simulink model "system_control"  (R2021a)
settings: Solver=FixedStepAuto  StartTime=0.0  StopTime=60  FixedStep=0.02  RelTol=1e-3
undefined symbols (not defined in the file): alpha, tau_d, v, yaw
libraries: simulink x2
(part 1 of 2)
settings Model: Creator=frede  LastModifiedBy=frede
settings DataIOCC: ReturnWorkspaceOutputs=off

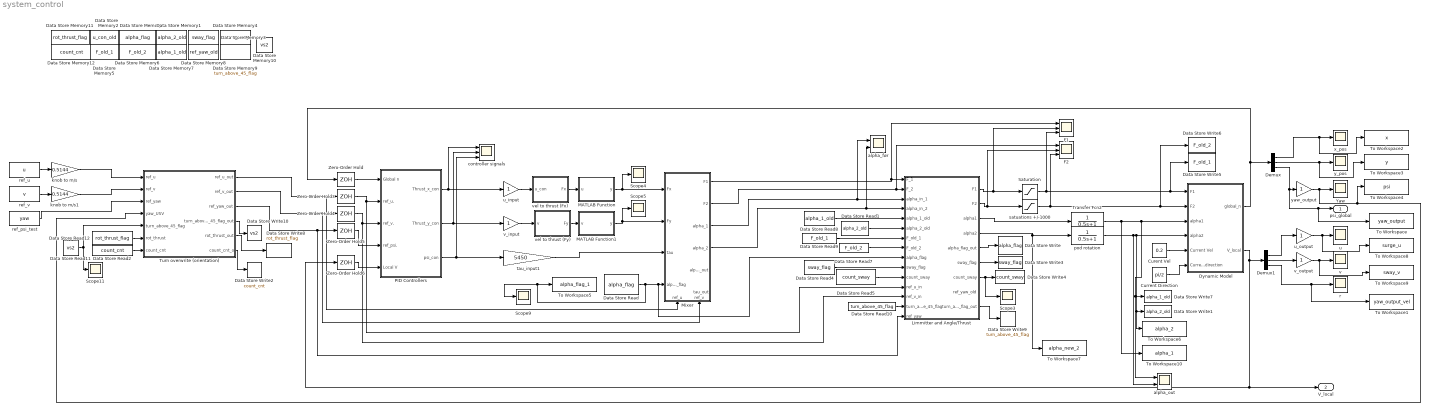
== system system_control ==
  Curent Vel : Constant  Value=0.2
  Current Direction : Constant  Value=pi/2
  Data Store Memory : DataStoreMemory  DataStoreName=alpha_flag  ReadBeforeWriteMsg=warning  WriteAfterWriteMsg=warning  WriteAfterReadMsg=warning  ShowAdditionalParam=off
  Data Store Memory1 : DataStoreMemory  DataStoreName=alpha_2_old  ReadBeforeWriteMsg=warning  WriteAfterWriteMsg=warning  WriteAfterReadMsg=warning  ShowAdditionalParam=off
  Data Store Memory10 : DataStoreMemory  DataStoreName=vs2  ReadBeforeWriteMsg=warning  WriteAfterWriteMsg=warning  WriteAfterReadMsg=warning  ShowAdditionalParam=off
  Data Store Memory11 : DataStoreMemory  DataStoreName=rot_thrust_flag  ReadBeforeWriteMsg=warning  WriteAfterWriteMsg=warning  WriteAfterReadMsg=warning  ShowAdditionalParam=off
  Data Store Memory12 : DataStoreMemory  DataStoreName=count_cnt  ReadBeforeWriteMsg=warning  WriteAfterWriteMsg=warning  WriteAfterReadMsg=warning  ShowAdditionalParam=off
  Data Store Memory2 : DataStoreMemory  DataStoreName=u_con_old  ReadBeforeWriteMsg=warning  WriteAfterWriteMsg=warning  WriteAfterReadMsg=warning  ShowAdditionalParam=off
  Data Store Memory3 : DataStoreMemory  DataStoreName=sway_flag  ReadBeforeWriteMsg=warning  WriteAfterWriteMsg=warning  WriteAfterReadMsg=warning  ShowAdditionalParam=off
  Data Store Memory4 : DataStoreMemory  DataStoreName=count_sway  ReadBeforeWriteMsg=warning  WriteAfterWriteMsg=warning  WriteAfterReadMsg=warning  ShowAdditionalParam=off
  Data Store Memory5 : DataStoreMemory  DataStoreName=F_old_1  ReadBeforeWriteMsg=warning  WriteAfterWriteMsg=warning  WriteAfterReadMsg=warning  ShowAdditionalParam=off
  Data Store Memory6 : DataStoreMemory  DataStoreName=F_old_2  ReadBeforeWriteMsg=warning  WriteAfterWriteMsg=warning  WriteAfterReadMsg=warning  ShowAdditionalParam=off
  Data Store Memory7 : DataStoreMemory  DataStoreName=alpha_1_old  ReadBeforeWriteMsg=warning  WriteAfterWriteMsg=warning  WriteAfterReadMsg=warning  ShowAdditionalParam=off
  Data Store Memory8 : DataStoreMemory  DataStoreName=ref_yaw_old  ReadBeforeWriteMsg=warning  WriteAfterWriteMsg=warning  WriteAfterReadMsg=warning  ShowAdditionalParam=off
  Data Store Memory9 : DataStoreMemory  DataStoreName=turn_above_45_flag  ReadBeforeWriteMsg=warning  WriteAfterWriteMsg=warning  WriteAfterReadMsg=warning  ShowAdditionalParam=off
  Data Store Read : DataStoreRead  DataStoreName=alpha_flag  IndexOptions=Index vector (dialog)  Indices=1  OutputSizes=1
  Data Store Read1 : DataStoreRead  DataStoreName=alpha_2_old  IndexOptions=Index vector (dialog)  Indices=1  OutputSizes=1
  Data Store Read10 : DataStoreRead  DataStoreName=turn_above_45_flag  IndexOptions=Index vector (dialog)  Indices=1  OutputSizes=1
  Data Store Read11 : DataStoreRead  DataStoreName=vs2  IndexOptions=Index vector (dialog)  Indices=1  OutputSizes=1
  Data Store Read12 : DataStoreRead  DataStoreName=rot_thrust_flag  IndexOptions=Index vector (dialog)  Indices=1  OutputSizes=1
  Data Store Read2 : DataStoreRead  DataStoreName=count_cnt  IndexOptions=Index vector (dialog)  Indices=1  OutputSizes=1
  Data Store Read4 : DataStoreRead  DataStoreName=sway_flag  IndexOptions=Index vector (dialog)  Indices=1  OutputSizes=1
  Data Store Read5 : DataStoreRead  DataStoreName=count_sway  IndexOptions=Index vector (dialog)  Indices=1  OutputSizes=1
  Data Store Read7 : DataStoreRead  DataStoreName=F_old_2  IndexOptions=Index vector (dialog)  Indices=1  OutputSizes=1
  Data Store Read8 : DataStoreRead  DataStoreName=alpha_1_old  IndexOptions=Index vector (dialog)  Indices=1  OutputSizes=1
  Data Store Read9 : DataStoreRead  DataStoreName=F_old_1  IndexOptions=Index vector (dialog)  Indices=1  OutputSizes=1
  Data Store Write : DataStoreWrite  DataStoreName=alpha_flag  IndexOptions=Index vector (dialog)  Indices=1  OutputSizes=1
  Data Store Write1 : DataStoreWrite  DataStoreName=alpha_2_old  IndexOptions=Index vector (dialog)  Indices=1  OutputSizes=1
  Data Store Write10 : DataStoreWrite  DataStoreName=vs2  IndexOptions=Index vector (dialog)  Indices=1  OutputSizes=1
  Data Store Write2 : DataStoreWrite  DataStoreName=count_cnt  IndexOptions=Index vector (dialog)  Indices=1  OutputSizes=1
  Data Store Write3 : DataStoreWrite  DataStoreName=sway_flag  IndexOptions=Index vector (dialog)  Indices=1  OutputSizes=1
  Data Store Write4 : DataStoreWrite  DataStoreName=count_sway  IndexOptions=Index vector (dialog)  Indices=1  OutputSizes=1
  Data Store Write5 : DataStoreWrite  DataStoreName=F_old_1  IndexOptions=Index vector (dialog)  Indices=1  OutputSizes=1
  Data Store Write6 : DataStoreWrite  DataStoreName=F_old_2  IndexOptions=Index vector (dialog)  Indices=1  OutputSizes=1
  Data Store Write7 : DataStoreWrite  DataStoreName=alpha_1_old  IndexOptions=Index vector (dialog)  Indices=1  OutputSizes=1
  Data Store Write8 : DataStoreWrite  DataStoreName=rot_thrust_flag  IndexOptions=Index vector (dialog)  Indices=1  OutputSizes=1
  Data Store Write9 : DataStoreWrite  DataStoreName=turn_above_45_flag  IndexOptions=Index vector (dialog)  Indices=1  OutputSizes=1
  Demux : Demux  Outputs=3
  Demux1 : Demux  Outputs=3
  Dynamic Model : Subsystem
  F1 : Scope  NumInputPorts=3
  F2 : Scope  NumInputPorts=3
  "Limmitter and Angle/Thrust " : MATLAB Function  TreatAsAtomicUnit=on
  MATLAB Function : MATLAB Function  TreatAsAtomicUnit=on
  MATLAB Function1 : MATLAB Function  TreatAsAtomicUnit=on
  Mixer : Subsystem
      settings: PortSchema="{\"entries\":[{\"content\":{\"sides\":[{\"content\":{\"connectorIds\":[\"In1\",\"In2\",\"In3\",\"In4\"]},\"type\":\"ConnectorPlacement.EquallySpacedRectSide\",\"uuid\":\"7188d02b-cfcc-47db-af94-18894173419c\"},{\"content\":{\"connectorIds\":[\"Out1\",\"Out2\",\"Out3\",\"Out4\",\"Out5\",\"Out6\"],\"side\":\"RIGHT\"},\"type\":\"ConnectorPlacement.EquallySpacedRectSide\",\"uuid\":\"02945fdb-bbe4-4a20-85bf-b896b72802e6\"},{\"content\":{\"connectorIds\":[],\"side\":\"TOP\"},\"type\":\"ConnectorPlacement.EquallySpacedRectSide\",\"uuid\":\"f10c450a-087c-46ba-bf6c-a28873fc7004\"},{\"content\":{\"connectorIds\":[\"In5\",\"In6\"],\"side\":\"BOTTOM\"},\"type\":\"ConnectorPlacement.EquallySpacedRectSide\",\"uuid\":\"e6b9d579-da5b-4e58-b3fd-82de45e53b4e\"}]},\"type\":\"ConnectorPlacement.EquallySpacedConnector\",\"uuid\":\"11fe65e6-3ea5-4662-a95f-67184bab7731\"}],\"packageUris\":[\"http://schema.mathworks.com/mf0/Connector/R2020b\"],\"version\":\"1.0\"}"
  PID Controllers : Subsystem
  Saturation : Saturate  UpperLimit=1000  LowerLimit=-1000
  Scope{3..5,9,11} (5 alike) : Scope
  To Workspace : ToWorkspace  VariableName=yaw_output  SaveFormat=Timeseries  SampleTime=-1
  To Workspace1 : ToWorkspace  VariableName=yaw_output_vel  SaveFormat=Timeseries  SampleTime=-1
  To Workspace10 : ToWorkspace  VariableName=alpha_1  SaveFormat=Timeseries  SampleTime=-1
  To Workspace2 : ToWorkspace  VariableName=x  SaveFormat=Timeseries  SampleTime=-1
  To Workspace3 : ToWorkspace  VariableName=y  SaveFormat=Timeseries  SampleTime=-1
  To Workspace4 : ToWorkspace  VariableName=psi  SaveFormat=Timeseries  SampleTime=-1
  To Workspace5 : ToWorkspace  VariableName=alpha_flag_1  SaveFormat=Timeseries  SampleTime=-1
  To Workspace6 : ToWorkspace  VariableName=alpha_2  SaveFormat=Timeseries  SampleTime=-1
  To Workspace7 : ToWorkspace  VariableName=alpha_new_2  SaveFormat=Timeseries  SampleTime=-1
  To Workspace8 : ToWorkspace  VariableName=surge_u  SaveFormat=Timeseries  SampleTime=-1
  To Workspace9 : ToWorkspace  VariableName=sway_v  SaveFormat=Timeseries  SampleTime=-1
  Transfer Fcn2 : TransferFcn  Denominator=[0.5 1]
  Turn overwrite (orientation) : MATLAB Function  TreatAsAtomicUnit=on
  Yaw : Scope
  Zero-Order Hold{,3..6} (5 alike) : ZeroOrderHold  SampleTime=1/10
  alpha_før : Scope  NumInputPorts=2
  alpha_out : Scope  NumInputPorts=2
  controller signals : Scope  NumInputPorts=3
  knob to m/s : Gain  Gain=0.5144
  knob to m/s1 : Gain  Gain=0.5144
  pod rotation : TransferFcn  Denominator=[0.5 1]
  r : Scope
  ref_psi_test : Constant  Value=yaw
  ref_u : Constant  Value=u
  ref_v : Constant  Value=v
  "satuations +/-1000 " : Saturate  UpperLimit=1000  LowerLimit=-1000
  tau_input1 : Gain  Gain=5450
  u : Scope
  u_input : Gain
  u_output : Gain
  v : Scope
  v_input : Gain
  v_output : Gain
  vel to thrust (Fx) : MATLAB Function  TreatAsAtomicUnit=on
  vel to thrust (Fy) : MATLAB Function  TreatAsAtomicUnit=on
  x_pos : Scope
  y_pos : Scope
  yaw_output : Gain
  psi_global : Outport
  V_local : Outport  Port=2
  wires:
  vel to thrust (Fx)/1(Fx) -> MATLAB Function/1(u)
  Demux1/3 -> r/1, To Workspace1/1
  "Limmitter and Angle/Thrust "/2(F2) -> "satuations +/-1000 "/1, F2/2
  Mixer/1(F1) -> F1/1, "Limmitter and Angle/Thrust "/1(F_1)
  v_input/1 -> vel to thrust (Fy)/1(v)
  Mixer/4(alpha_2) -> alpha_før/2, "Limmitter and Angle/Thrust "/4(alpha_in_2)
  Demux1/2 -> v_output/1
  Mixer/2(F2) -> F2/1, "Limmitter and Angle/Thrust "/2(F_2)
  "Limmitter and Angle/Thrust "/3(alpha1) -> Transfer Fcn2/1
  u_input/1 -> vel to thrust (Fx)/1(u_con)
  MATLAB Function1/1(y) -> Scope5/1, Mixer/2(Fy)
  Mixer/3(alpha_1) -> alpha_før/1, "Limmitter and Angle/Thrust "/3(alpha_in_1)
  "Limmitter and Angle/Thrust "/1(F1) -> F1/2, Saturation/1
  Demux/2 -> To Workspace3/1, y_pos/1
  "satuations +/-1000 "/1 -> Data Store Write6/1, Dynamic Model/2(F2), F2/3
  Demux1/1 -> u_output/1
  Transfer Fcn2/1 -> To Workspace10/1, Data Store Write7/1, alpha_out/1, Dynamic Model/3(alpha1)
  Dynamic Model/1(global_n) -> Zero-Order Hold/1, Demux/1
  "Limmitter and Angle/Thrust "/4(alpha2) -> To Workspace7/1, pod rotation/1
  Demux/1 -> To Workspace2/1, x_pos/1
  v_output/1 -> To Workspace9/1, v/1
  Saturation/1 -> Data Store Write5/1, Dynamic Model/1(F1), F1/3
  ref_v/1 -> knob to m/s1/1
  Demux/3 -> yaw_output/1, To Workspace/1, psi_global/1
  MATLAB Function/1(y) -> Mixer/1(Fx), Scope4/1
  yaw_output/1 -> Yaw/1, Turn overwrite (orientation)/4(yaw_USV), To Workspace4/1
  vel to thrust (Fy)/1(Fy) -> MATLAB Function1/1(v)
  Turn overwrite (orientation)/3(ref_yaw_out) -> "Limmitter and Angle/Thrust "/15(ref_yaw), Zero-Order Hold5/1
  Curent Vel/1 -> Dynamic Model/5(Current Vel)
  Current Direction/1 -> Dynamic Model/6(Current direction)
  ref_u/1 -> knob to m/s/1
  Turn overwrite (orientation)/2(ref_v_out) -> Zero-Order Hold4/1, Mixer/6(ref_v)
  "Limmitter and Angle/Thrust "/5(alpha_flag_out) -> Data Store Write/1
  Data Store Read1/1 -> "Limmitter and Angle/Thrust "/6(alpha_2_old)
  Data Store Read/1 -> Scope9/1, To Workspace5/1, "Limmitter and Angle/Thrust "/9(alpha_flag), Mixer/4(alpha_flag)
  Zero-Order Hold/1 -> PID Controllers/1(Global n)
  Turn overwrite (orientation)/1(ref_u_out) -> Zero-Order Hold3/1, Mixer/5(ref_u)
  Dynamic Model/2(V_local) -> V_local/1, Zero-Order Hold6/1, Demux1/1
  Zero-Order Hold3/1 -> "Limmitter and Angle/Thrust "/12(ref_u_in), PID Controllers/2(ref_u.)
  Zero-Order Hold4/1 -> "Limmitter and Angle/Thrust "/13(ref_v_in), PID Controllers/3(ref_v.)
  Zero-Order Hold5/1 -> PID Controllers/4(ref_psi.)
  Zero-Order Hold6/1 -> PID Controllers/5(Local V)
  "Limmitter and Angle/Thrust "/6(sway_flag) -> Data Store Write3/1
  Data Store Read5/1 -> "Limmitter and Angle/Thrust "/11("count_sway ")
  tau_input1/1 -> Mixer/3(tau)
  Data Store Read8/1 -> "Limmitter and Angle/Thrust "/5(alpha_1_old)
  Data Store Read7/1 -> "Limmitter and Angle/Thrust "/8(F_old_2)
  Data Store Read9/1 -> "Limmitter and Angle/Thrust "/7(F_old_1)
  Data Store Read4/1 -> "Limmitter and Angle/Thrust "/10("sway_flag ")
  "Limmitter and Angle/Thrust "/7(count_sway) -> Scope3/1, Data Store Write4/1
  Data Store Read10/1 -> "Limmitter and Angle/Thrust "/14(turn_above_45_flag)
  "Limmitter and Angle/Thrust "/9(turn_above_45_flag_out) -> Data Store Write9/1
  Turn overwrite (orientation)/4(turn_above_45_flag_out) -> Data Store Write10/1
  Data Store Read11/1 -> Turn overwrite (orientation)/5(turn_above_45_flag), Scope11/1
  PID Controllers/2(Thrust_y_con) -> v_input/1, controller signals/2
  PID Controllers/1(Thrust_x_con) -> u_input/1, controller signals/1
  PID Controllers/3(psi_con) -> tau_input1/1, controller signals/3
  Data Store Read12/1 -> Turn overwrite (orientation)/6(rot_thrust)
  Turn overwrite (orientation)/5(rot_thrust_out) -> Data Store Write8/1
  knob to m/s/1 -> Turn overwrite (orientation)/1(ref_u)
  knob to m/s1/1 -> Turn overwrite (orientation)/2(ref_v)
  ref_psi_test/1 -> Turn overwrite (orientation)/3(ref_yaw)
  pod rotation/1 -> Dynamic Model/4(alpha2), To Workspace6/1, Data Store Write1/1, alpha_out/2
  Turn overwrite (orientation)/6(count_cnt_o) -> Data Store Write2/1
  Data Store Read2/1 -> Turn overwrite (orientation)/7(count_cnt)
  u_output/1 -> To Workspace8/1, u/1

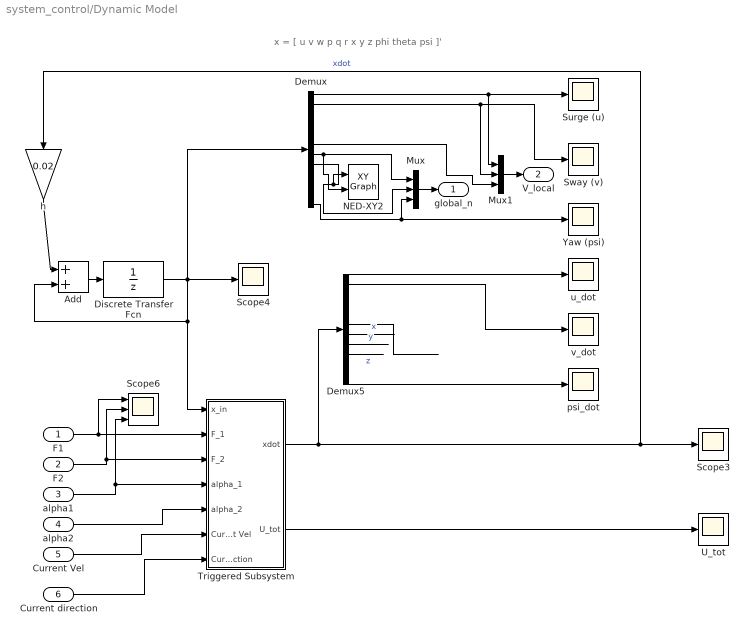
== system system_control/Dynamic Model ==
  note: x = [ u v w p q r x y z phi theta psi ]'
  F1 : Inport
  F2 : Inport  Port=2
  alpha1 : Inport  Port=3
  alpha2 : Inport  Port=4
  Current Vel : Inport  Port=5
  Current direction : Inport  Port=6
  Add : Sum
  Demux : Demux  Outputs=12
  Demux5 : Demux  Outputs=12
  Discrete Transfer Fcn : DiscreteTransferFcn  Denominator=[ 1 0]  SampleTime=0.02
  Mux : Mux  Inputs=3
  Mux1 : Mux  Inputs=3
  NED-XY2 : simulink/Sinks/XY Graph  xmin=-10  xmax=100  ymin=-10  ymax=100  st=-1
  Scope3 : Scope
  Scope4 : Scope
  Scope6 : Scope  NumInputPorts=3
  Surge (u) : Scope
  Sway (v) : Scope
  Triggered Subsystem : Subsystem  TreatAsAtomicUnit=on
  U_tot : Scope
  Yaw (psi) : Scope
  h : Gain  Gain=0.02
  psi_dot : Scope
  u_dot : Scope
  v_dot : Scope
  global_n : Outport
  V_local : Outport  Port=2
  wires:
  F1/1 -> Scope6/1, Triggered Subsystem/2(F_1)
  F2/1 -> Scope6/2, Triggered Subsystem/3(F_2)
  alpha1/1 -> Scope6/3, Triggered Subsystem/4(alpha_1)
  alpha2/1 -> Triggered Subsystem/5(alpha_2)
  h/1 -> Add/1
  Add/1 -> Discrete Transfer Fcn/1
  Triggered Subsystem/1(xdot) -> Demux5/1, Scope3/1, h/1  "xdot"
  Triggered Subsystem/2(U_tot) -> U_tot/1
  Demux/8 -> Mux/2, NED-XY2/1
  Demux/7 -> NED-XY2/2, Mux/1
  Discrete Transfer Fcn/1 -> Scope4/1, Demux/1, Add/2, Triggered Subsystem/1(x_in)
  Demux/1 -> Surge (u)/1, Mux1/1
  Demux/12 -> Mux/3, Yaw (psi)/1
  Demux/2 -> Mux1/2, Sway (v)/1
  Mux/1 -> global_n/1
  Demux5/12 -> psi_dot/1
  Demux5/2 -> v_dot/1
  Demux5/1 -> u_dot/1
  Demux5/9 -> ?  "z"
  Demux5/7 -> ?  "x"
  Demux5/8 -> ?  "y"
  Mux1/1 -> V_local/1
  Demux5/6 -> ?
  Demux/6 -> Mux1/3
  Current Vel/1 -> Triggered Subsystem/6(Current Vel)
  Current direction/1 -> Triggered Subsystem/7(Current Direction)

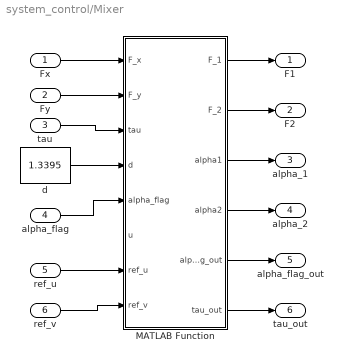
== system system_control/Mixer ==
  Fx : Inport
  Fy : Inport  Port=2
  tau : Inport  Port=3
  alpha_flag : Inport  Port=4
  ref_u : Inport  Port=5
  ref_v : Inport  Port=6
  MATLAB Function : MATLAB Function  TreatAsAtomicUnit=on
  d : Constant  Value=1.3395
  F1 : Outport
  F2 : Outport  Port=2
  alpha_1 : Outport  Port=3
  alpha_2 : Outport  Port=4
  alpha_flag_out : Outport  Port=5
  tau_out : Outport  Port=6
  wires:
  d/1 -> MATLAB Function/4(d)
  MATLAB Function/1(F_1) -> F1/1
  Fx/1 -> MATLAB Function/1(F_x)
  Fy/1 -> MATLAB Function/2(F_y)
  tau/1 -> MATLAB Function/3(tau)
  MATLAB Function/2(F_2) -> F2/1
  MATLAB Function/3(alpha1) -> alpha_1/1
  MATLAB Function/4(alpha2) -> alpha_2/1
  alpha_flag/1 -> MATLAB Function/5(alpha_flag)
  MATLAB Function/5(alpha_flag_out) -> alpha_flag_out/1
  ref_u/1 -> MATLAB Function/7(ref_u)
  ref_v/1 -> MATLAB Function/8(ref_v)
  MATLAB Function/6(tau_out) -> tau_out/1

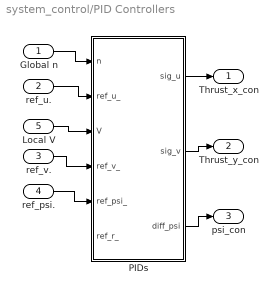
== system system_control/PID Controllers ==
  Global n : Inport
  ref_u. : Inport  Port=2
  ref_v. : Inport  Port=3
  ref_psi. : Inport  Port=4
  Local V : Inport  Port=5
  PIDs : Subsystem
  Thrust_x_con : Outport
  Thrust_y_con : Outport  Port=2
  psi_con : Outport  Port=3
  wires:
  Global n/1 -> PIDs/1(n)
  ref_v./1 -> PIDs/4(ref_v_)
  PIDs/3(diff_psi) -> psi_con/1
  PIDs/1(sig_u) -> Thrust_x_con/1
  PIDs/2(sig_v) -> Thrust_y_con/1
  ref_u./1 -> PIDs/2(ref_u_)
  Local V/1 -> PIDs/3(V)
  ref_psi./1 -> PIDs/5(ref_psi_)

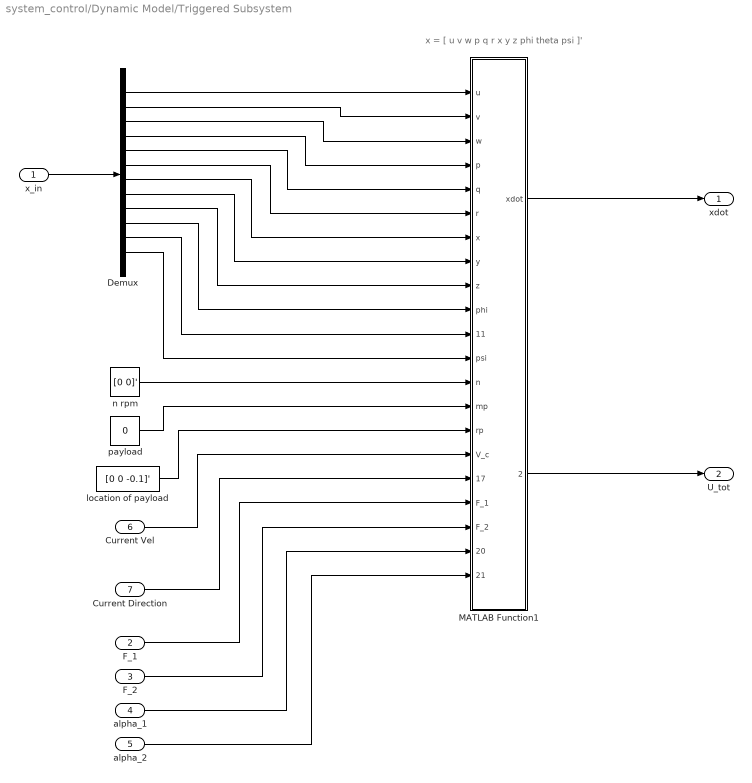
== system system_control/Dynamic Model/Triggered Subsystem ==
  note: x = [ u v w p q r x y z phi theta psi ]'
  x_in : Inport
  F_1 : Inport  Port=2
  F_2 : Inport  Port=3
  alpha_1 : Inport  Port=4
  alpha_2 : Inport  Port=5
  Current Vel : Inport  Port=6
  Current Direction : Inport  Port=7
  Demux : Demux  Outputs=12
  MATLAB Function1 : MATLAB Function  TreatAsAtomicUnit=on
  location of payload : Constant  Value=[0 0 -0.1]'
  n rpm : Constant  Value=[0 0]'
  payload : Constant  Value=0
  xdot : Outport
  U_tot : Outport  Port=2
  wires:
  F_1/1 -> MATLAB Function1/18(F_1)
  F_2/1 -> MATLAB Function1/19(F_2)
  alpha_1/1 -> MATLAB Function1/20(alpha_1)
  alpha_2/1 -> MATLAB Function1/21(alpha_2)
  location of payload/1 -> MATLAB Function1/15(rp)
  payload/1 -> MATLAB Function1/14(mp)
  Current Vel/1 -> MATLAB Function1/16(V_c)
  Current Direction/1 -> MATLAB Function1/17(beta_c)
  n rpm/1 -> MATLAB Function1/13(n)
  x_in/1 -> Demux/1
  MATLAB Function1/2(U_tot) -> U_tot/1
  MATLAB Function1/1(xdot) -> xdot/1
  Demux/1 -> MATLAB Function1/1(u)
  Demux/2 -> MATLAB Function1/2(v)
  Demux/3 -> MATLAB Function1/3(w)
  Demux/4 -> MATLAB Function1/4(p)
  Demux/5 -> MATLAB Function1/5(q)
  Demux/6 -> MATLAB Function1/6(r)
  Demux/7 -> MATLAB Function1/7(x)
  Demux/8 -> MATLAB Function1/8(y)
  Demux/9 -> MATLAB Function1/9(z)
  Demux/10 -> MATLAB Function1/10(phi)
  Demux/11 -> MATLAB Function1/11(theta)
  Demux/12 -> MATLAB Function1/12(psi)

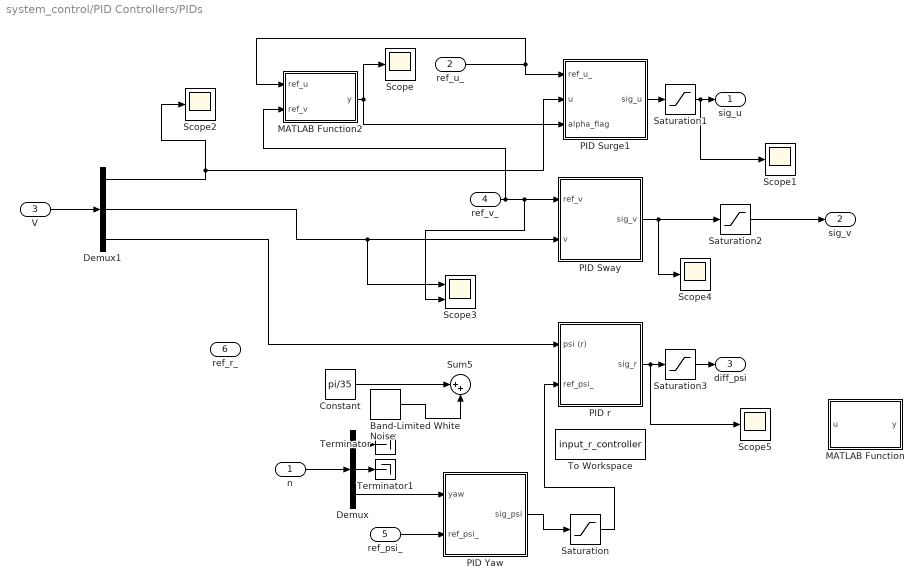
== system system_control/PID Controllers/PIDs ==
  n : Inport
  ref_u_ : Inport  Port=2
  V : Inport  Port=3
  ref_v_ : Inport  Port=4
  ref_psi_ : Inport  Port=5
  ref_r_ : Inport  Port=6
  Band-Limited White Noise : simulink/Sources/Band-Limited White Noise  Cov=[0.01]  Ts=0.1  seed=[23341]
  Constant : Constant  Value=pi/35
  Demux : Demux  Outputs=3
  Demux1 : Demux  Outputs=3
  MATLAB Function : MATLAB Function  TreatAsAtomicUnit=on
  MATLAB Function2 : MATLAB Function  TreatAsAtomicUnit=on
  PID Surge1 : Subsystem
  PID Sway : Subsystem
  PID Yaw : Subsystem
  PID r : Subsystem
  Saturation : Saturate  UpperLimit=0.18  LowerLimit=-0.18
  Saturation1 : Saturate  UpperLimit=20  LowerLimit=-20
  Saturation2 : Saturate  UpperLimit=20  LowerLimit=-20
  Saturation3 : Saturate  UpperLimit=2  LowerLimit=-2
  Scope{,1..2,4..5} (5 alike) : Scope
  Scope3 : Scope  NumInputPorts=2
  Sum5 : Sum  Inputs=|++
  Terminator : Terminator
  Terminator1 : Terminator
  To Workspace : ToWorkspace  VariableName=input_r_controller  SaveFormat=Timeseries  SampleTime=-1
  sig_u : Outport
  sig_v : Outport  Port=2
  diff_psi : Outport  Port=3
  wires:
  n/1 -> Demux/1
  Demux/3 -> PID Yaw/1(yaw)
  Demux/1 -> Terminator/1
  Demux/2 -> Terminator1/1
  Demux1/3 -> PID r/1(psi (r))
  V/1 -> Demux1/1
  ref_u_/1 -> PID Surge1/1(ref_u_), MATLAB Function2/1(ref_u)
  Demux1/1 -> Scope2/1, PID Surge1/2(u)
  ref_v_/1 -> Scope3/2, PID Sway/1(ref_v), MATLAB Function2/2(ref_v)
  Band-Limited White Noise/1 -> Sum5/2
  Constant/1 -> Sum5/1
  PID Sway/1(sig_v) -> Scope4/1, Saturation2/1
  PID r/1(sig_r) -> Scope5/1, Saturation3/1
  ref_psi_/1 -> PID Yaw/2(ref_psi_)
  PID Yaw/1(sig_psi) -> Saturation/1
  MATLAB Function2/1(y) -> PID Surge1/3(alpha_flag), Scope/1
  Saturation/1 -> PID r/2(ref_psi_)
  Demux1/2 -> Scope3/1, PID Sway/2(v)
  PID Surge1/1(sig_u) -> Saturation1/1
  Saturation1/1 -> Scope1/1, sig_u/1
  Saturation2/1 -> sig_v/1
  Saturation3/1 -> diff_psi/1

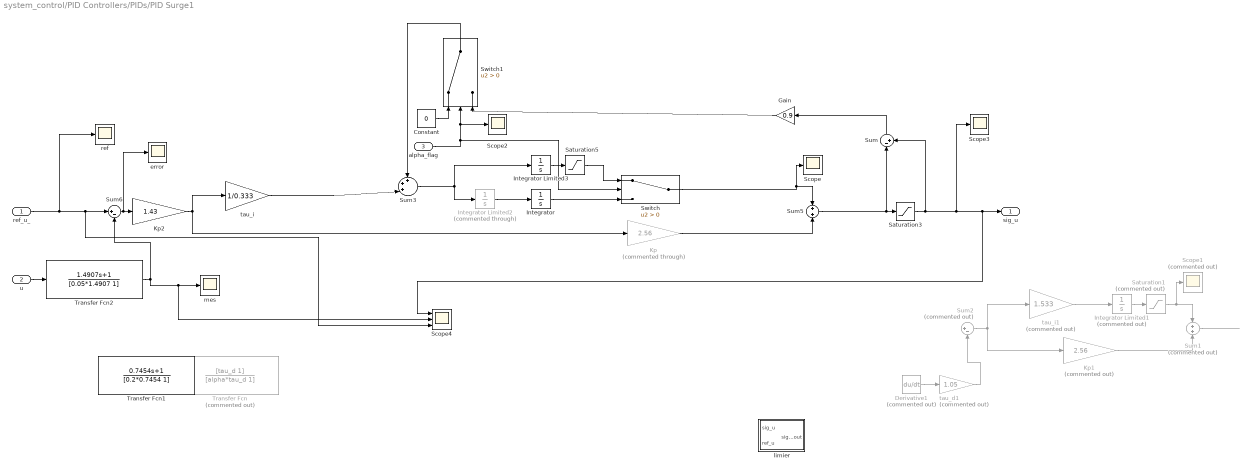
== system system_control/PID Controllers/PIDs/PID Surge1 ==
  ref_u_ : Inport
  u : Inport  Port=2
  alpha_flag : Inport  Port=3
  Constant : Constant  Value=0
  Derivative1 : Derivative  Commented=on
  Gain : Gain  Gain=0.9
  Integrator : Integrator
  Integrator Limited1 : Integrator  Commented=on  LimitOutput=on  UpperSaturationLimit=1  LowerSaturationLimit=-1
  Integrator Limited2 : Integrator  Commented=through  LimitOutput=on  UpperSaturationLimit=0.5144  LowerSaturationLimit=-0.5144
  Integrator Limited3 : Integrator  LimitOutput=on  UpperSaturationLimit=0.2  LowerSaturationLimit=-0.2
  Kp : Gain  Commented=through  Gain=2.56
  Kp1 : Gain  Commented=on  Gain=2.56
  Kp2 : Gain  Gain=1.43
  Saturation1 : Saturate  Commented=on  UpperLimit=5  LowerLimit=-5
  Saturation3 : Saturate  UpperLimit=8*0.54133  LowerLimit=-8*0.54133
  Saturation5 : Saturate  UpperLimit=0  LowerLimit=0
  Scope : Scope
  Scope1 : Scope  Commented=on
  Scope2 : Scope
  Scope3 : Scope
  Scope4 : Scope  NumInputPorts=3
  Sum : Sum  Inputs=|-+
  Sum1 : Sum  Commented=on
  Sum2 : Sum  Commented=on  Inputs=|+-
  Sum3 : Sum  Inputs=+++|
  Sum5 : Sum
  Sum6 : Sum  Inputs=|+-
  Switch : Switch  Criteria=u2 > Threshold
  Switch1 : Switch  Criteria=u2 > Threshold
  Transfer Fcn : TransferFcn  Commented=on  Numerator=[tau_d 1]  Denominator=[alpha*tau_d 1]
  Transfer Fcn1 : TransferFcn  Numerator=[0.7454 1]  Denominator=[0.2*0.7454 1]
  Transfer Fcn2 : TransferFcn  Numerator=[1.4907 1]  Denominator=[0.05*1.4907 1]
  error : Scope
  limier : MATLAB Function  TreatAsAtomicUnit=on
  mes : Scope
  ref : Scope
  tau_d1 : Gain  Commented=on  Gain=1.05
  tau_i : Gain  Gain=1/0.333
  tau_i1 : Gain  Commented=on  Gain=1.533
  sig_u : Outport
  wires:
  Transfer Fcn2/1 -> Sum6/2, Scope4/2, mes/1
  Kp/1 -> Sum5/2
  Sum6/1 -> error/1, Kp2/1
  u/1 -> Transfer Fcn2/1
  tau_i/1 -> Sum3/3
  Switch/1 -> Sum5/1, Scope/1
  ? -> Sum2/1
  Sum2/1 -> tau_i1/1, Kp1/1
  Kp1/1 -> Sum1/2
  Derivative1/1 -> tau_d1/1
  Saturation1/1 -> Sum1/1, Scope1/1
  ? -> Derivative1/1
  tau_d1/1 -> Sum2/2
  Integrator Limited1/1 -> Saturation1/1
  Sum1/1 -> ?
  tau_i1/1 -> Integrator Limited1/1
  Sum5/1 -> Sum/1, Saturation3/1
  Sum/1 -> Gain/1
  Kp2/1 -> tau_i/1, Kp/1
  Switch1/1 -> Sum3/1
  Integrator/1 -> Switch/3
  Integrator Limited3/1 -> Saturation5/1
  Saturation5/1 -> Switch/1
  alpha_flag/1 -> Scope2/1, Switch1/2, Switch/2
  Gain/1 -> Switch1/3
  Constant/1 -> Switch1/1
  Sum3/1 -> Integrator Limited2/1, Integrator Limited3/1
  Saturation3/1 -> Scope3/1, Scope4/1, sig_u/1, Sum/2
  Integrator Limited2/1 -> Integrator/1
  ref_u_/1 -> ref/1, Scope4/3, Sum6/1

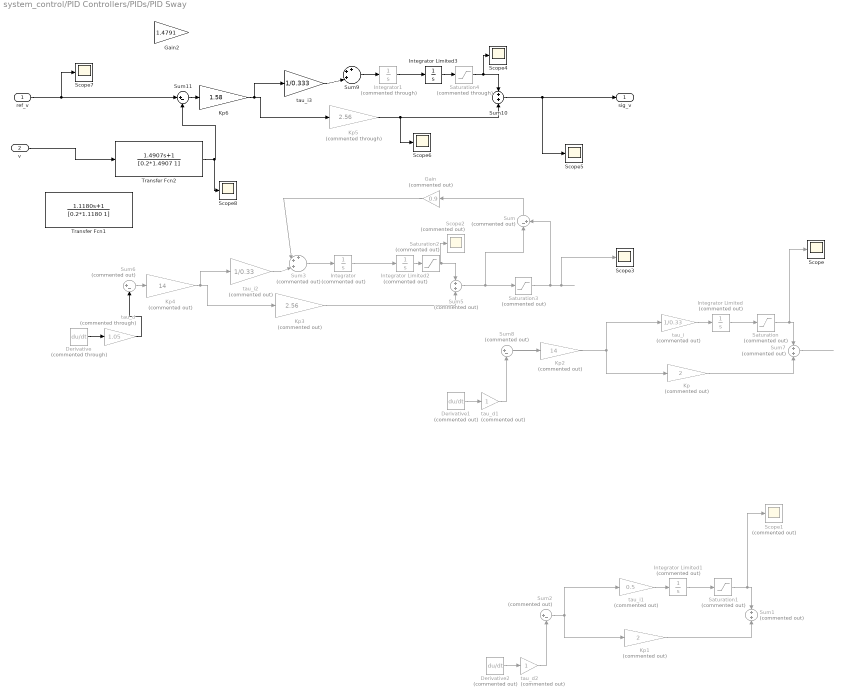
== system system_control/PID Controllers/PIDs/PID Sway ==
  ref_v : Inport
  v : Inport  Port=2
  Derivative : Derivative  Commented=through
  Derivative1 : Derivative  Commented=on
  Derivative2 : Derivative  Commented=on
  Gain : Gain  Commented=on  Gain=0.9
  Gain2 : Gain  Gain=1.4791
  Integrator : Integrator  Commented=on
  Integrator Limited : Integrator  Commented=on  LimitOutput=on  UpperSaturationLimit=1  LowerSaturationLimit=-1
  Integrator Limited1 : Integrator  Commented=on  LimitOutput=on  UpperSaturationLimit=1  LowerSaturationLimit=-1
  Integrator Limited2 : Integrator  Commented=on  LimitOutput=on  UpperSaturationLimit=2  LowerSaturationLimit=-2
  Integrator Limited3 : Integrator  LimitOutput=on  UpperSaturationLimit=2*0.54133+0.5  LowerSaturationLimit=-2*0.54133-0.5
  Integrator1 : Integrator  Commented=through
  Kp : Gain  Commented=on  Gain=2
  Kp1 : Gain  Commented=on  Gain=2
  Kp2 : Gain  Commented=on  Gain=14
  Kp3 : Gain  Commented=on  Gain=2.56
  Kp4 : Gain  Commented=on  Gain=14
  Kp5 : Gain  Commented=through  Gain=2.56
  Kp6 : Gain  Gain=1.58
  Saturation : Saturate  Commented=on  UpperLimit=1  LowerLimit=-1
  Saturation1 : Saturate  Commented=on  UpperLimit=1  LowerLimit=-1
  Saturation2 : Saturate  Commented=on  UpperLimit=5  LowerLimit=-5
  Saturation3 : Saturate  Commented=on  UpperLimit=2  LowerLimit=-2
  Saturation4 : Saturate  Commented=through  UpperLimit=5  LowerLimit=-5
  Scope{,3..8} (7 alike) : Scope
  Scope1 : Scope  Commented=on
  Scope2 : Scope  Commented=on
  Sum : Sum  Commented=on  Inputs=|-+
  Sum1 : Sum  Commented=on
  Sum10 : Sum
  Sum11 : Sum  Inputs=|+-
  Sum2 : Sum  Commented=on  Inputs=|+-
  Sum3 : Sum  Commented=on  Inputs=+++|
  Sum5 : Sum  Commented=on
  Sum6 : Sum  Commented=on  Inputs=|+-
  Sum7 : Sum  Commented=on
  Sum8 : Sum  Commented=on  Inputs=|+-
  Sum9 : Sum  Inputs=+++|
  Transfer Fcn1 : TransferFcn  Numerator=[1.1180 1]  Denominator=[0.2*1.1180 1]
  Transfer Fcn2 : TransferFcn  Numerator=[1.4907 1]  Denominator=[0.2*1.4907 1]
  tau_d : Gain  Commented=through  Gain=1.05
  tau_d1 : Gain  Commented=on
  tau_d2 : Gain  Commented=on
  tau_i : Gain  Commented=on  Gain=1/0.33
  tau_i1 : Gain  Commented=on  Gain=0.5
  tau_i2 : Gain  Commented=on  Gain=1/0.33
  tau_i3 : Gain  Gain=1/0.333
  sig_v : Outport
  wires:
  Sum8/1 -> Kp2/1
  Kp/1 -> Sum7/2
  ? -> Sum8/1
  Integrator Limited/1 -> Saturation/1
  Derivative1/1 -> tau_d1/1
  Sum7/1 -> ?
  tau_d1/1 -> Sum8/2
  ? -> Derivative1/1
  tau_i/1 -> Integrator Limited/1
  Saturation/1 -> Scope/1, Sum7/1
  tau_i1/1 -> Integrator Limited1/1
  Derivative2/1 -> tau_d2/1
  Integrator Limited1/1 -> Saturation1/1
  Saturation1/1 -> Scope1/1, Sum1/1
  Sum2/1 -> tau_i1/1, Kp1/1
  Kp1/1 -> Sum1/2
  tau_d2/1 -> Sum2/2
  Kp2/1 -> tau_i/1, Kp/1
  Kp4/1 -> tau_i2/1, Kp3/1
  tau_d/1 -> Sum6/2
  Kp3/1 -> Sum5/2
  Integrator Limited2/1 -> Saturation2/1
  Saturation3/1 -> Scope3/1, Sum/2
  Gain/1 -> Sum3/2
  Derivative/1 -> tau_d/1
  Sum/1 -> Gain/1
  Sum3/1 -> Integrator/1
  Sum5/1 -> Saturation3/1, Sum/1
  ? -> Derivative/1
  Saturation2/1 -> Scope2/1, Sum5/1
  tau_i2/1 -> Sum3/3
  Sum6/1 -> Kp4/1
  ? -> Sum6/1
  Integrator/1 -> Integrator Limited2/1
  Transfer Fcn2/1 -> Scope8/1, Sum11/2
  Kp6/1 -> tau_i3/1, Kp5/1
  Kp5/1 -> Scope6/1, Sum10/2
  Integrator Limited3/1 -> Saturation4/1
  Saturation4/1 -> Sum10/1, Scope4/1
  tau_i3/1 -> Sum9/3
  Sum9/1 -> Integrator1/1
  Sum11/1 -> Kp6/1
  ref_v/1 -> Scope7/1, Sum11/1
  Integrator1/1 -> Integrator Limited3/1
  v/1 -> Transfer Fcn2/1
  Sum10/1 -> Scope5/1, sig_v/1

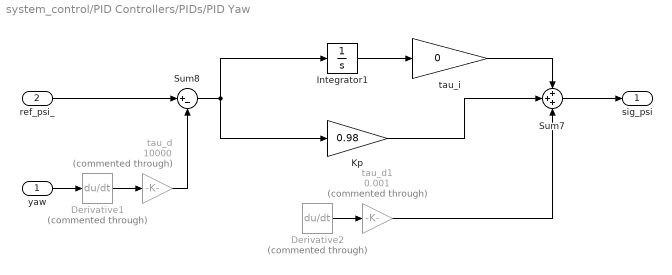
== system system_control/PID Controllers/PIDs/PID Yaw ==
  yaw : Inport
  ref_psi_ : Inport  Port=2
  Derivative1 : Derivative  Commented=through
  Derivative2 : Derivative  Commented=through
  Integrator1 : Integrator
  Kp : Gain  Gain=0.98
  Sum7 : Sum  Inputs=+++
  Sum8 : Sum  Inputs=|+-
  tau_d : Gain  Commented=through  Gain=10000
  tau_d1 : Gain  Commented=through  Gain=0.001
  tau_i : Gain  Gain=0
  sig_psi : Outport
  wires:
  Sum8/1 -> Kp/1, Integrator1/1
  Integrator1/1 -> tau_i/1
  Kp/1 -> Sum7/2
  ref_psi_/1 -> Sum8/1
  tau_i/1 -> Sum7/1
  Derivative1/1 -> tau_d/1
  Sum7/1 -> sig_psi/1
  tau_d/1 -> Sum8/2
  yaw/1 -> Derivative1/1
  Derivative2/1 -> tau_d1/1
  tau_d1/1 -> Sum7/3

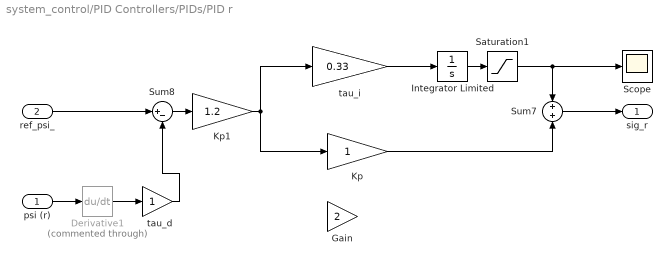
== system system_control/PID Controllers/PIDs/PID r ==
  psi (r) : Inport
  ref_psi_ : Inport  Port=2
  Derivative1 : Derivative  Commented=through
  Gain : Gain  Gain=2
  Integrator Limited : Integrator  LimitOutput=on  UpperSaturationLimit=0.2  LowerSaturationLimit=-0.2
  Kp : Gain
  Kp1 : Gain  Gain=1.2
  Saturation1 : Saturate  UpperLimit=10  LowerLimit=-10
  Scope : Scope
  Sum7 : Sum
  Sum8 : Sum  Inputs=|+-
  tau_d : Gain
  tau_i : Gain  Gain=0.33
  sig_r : Outport
  wires:
  Sum8/1 -> Kp1/1
  Kp/1 -> Sum7/2
  ref_psi_/1 -> Sum8/1
  Integrator Limited/1 -> Saturation1/1
  Derivative1/1 -> tau_d/1
  Sum7/1 -> sig_r/1
  tau_d/1 -> Sum8/2
  psi (r)/1 -> Derivative1/1
  tau_i/1 -> Integrator Limited/1
  Kp1/1 -> Kp/1, tau_i/1
  Saturation1/1 -> Scope/1, Sum7/1

== matlab function system_control/MATLAB Function ==
  data: u input; y output
function y = fcn(u)
   if(u == 0.0)
        out = 0.00000000000000000001;
    else
        out = u;
    
    end
    
    
  

y = out;

== matlab function system_control/PID Controllers/PIDs/MATLAB Function ==
  data: u input; y output
function y = fcn(u)

if (abs(u) < 0.02)
    y = 0;
else
    y=0;
end


y = u;

== matlab function system_control/Dynamic Model/Triggered Subsystem/MATLAB Function1 ==
  settings: updateMethod=DISCRETE
  data: u input; v input; w input; p input; q input; r input; x input; y input; z input; phi input; theta input; psi input; xdot output; n input; mp input; rp input; V_c input; beta_c input; F_1 input; F_2 input; alpha_1 input; alpha_2 input; U_tot output
function [xdot,U_tot] = otter(u, v, w, p, q, r, x, y, z, phi, theta, psi,n,mp,rp,V_c,beta_c,F_1,F_2,alpha_1,alpha_2)
% [xdot,U] = otter(x,n,mp,rp,V_c,beta_c) returns the speed U in m/s (optionally) 
% and the time derivative of the state vector: 
x = [u v w p q r x y z phi theta psi]'; 
% for the Maritime Robotics Otter USV, see www.maritimerobotics.com. 
% The length of the USV is L = 2.0 m, while the state vector is defined as:
%
%  u:     surge velocity          (m/s)
%  v:     sway velocity           (m/s)
%  w:     heave velocity          (m/s)
%  p:     roll velocity           (rad/s)
%  q:     pitch velocity          (rad/s)
%  r:     yaw velocity            (rad/s)
%  x:     position in x direction (m)
%  y:     position in y direction (m)
%  z:     position in z direction (m)
%  phi:   roll angle              (rad)
%  theta: pitch angle             (rad)
%  psi:   yaw angle               (rad)
%
% The other inputs are:
%
% n = [ n(1) n(2) ]' where
%    n(1): propeller shaft speed, left (rad/s)
%    n(2): propeller shaft speed, right (rad/s)
%
% mp = payload mass (kg), maximum 45 kg
%  rp = [xp, yp, zp]' (m) is the location of the payload w.r.t. the CO
%  V_c:     current speed (m/s)
%  beta_c:  current direction (rad)
%
% See, ExOtter.m and demoOtterUSVHeadingControl.slx
%
% Author:    Thor I. Fossen
% Date:      2019-07-17
% Revisions: 2021-04-25 added call to new function crossFlowDrag.m
%            2021-06-21 Munk moment in yaw is neglected
%            2021-07-22 Added a new state for the trim moment
%            2021-12-17 New method Xudot = -addedMassSurge(m,L,rho) 

% Check of input and state dimensions
if (length(x) ~= 12),error('x vector must have dimension 12!'); end
if (length(n) ~= 2),error('n vector must have dimension 2!'); end

% trim: theta = -7.5 deg corresponds to 13.5 cm less height aft maximum load
trim_setpoint = 280;

% trim_setpoint is a step input, which is filtered using the state trim_moment
persistent trim_moment;

if isempty(trim_moment)
   trim_moment = 0;
end



% Main data
g   = 9.81;           % acceleration of gravity (m/s^2)
rho = 1025;           % density of water
L = 6.969;            % length (m)
B = 3.465;            % beam (m)
m = 775;              % mass (kg)
rg = [0 0 -0.044]';   % CG for hull only (m)
% R44 = 0.4 * B;      % radii of gyrations (m)
% R55 = 0.25 * L;
% R66 = 0.25 * L;
R44 =  0.3171*B; %0.78934 * B;    %0.62879*B;  % radii of gyrations (m) 0.3171*B;
R55 = 0.18482 * L;    %0.24044*L; 
R66 = 0.23465 * L;    %0.38756*L; 
T_yaw = 1 ;%2.5;      % time constant in yaw (s)
Umax = 8 * 0.5144;    % max forward speed (m/s)


% Data for one pontoon
B_pont  = 0.696;     % beam of one pontoon (m)
y_pont  = 1.3395;    % distance from centerline to waterline area center (m)
Cw_pont = 0.75;      % waterline area coefficient (-)
%Cb_pont = 0.4;      % block coefficient, computed from m = 55 kg
Cb_pont = 0.375;     % overslagsberegning af Cb


%%%%%%%%%%%%%%%%%%%%%%%%%%%%%%%%%%%%%%%%%%%%%%%%%%%%%%%%%%%%%%%%%%%%%%%%%%

% State and current variables
nu = x(1:6);                                % velocities [u v w p q r]
nu1 = x(1:3);                               % velocities [u v w]
nu2 = x(4:6);                               % velocities [p q r]
eta = x(7:12);                              % positions [x y z phi theta psi ]
U = sqrt(nu(1)^2 + nu(2)^2 + nu(3)^2);      % speed
u_c = V_c * cos(beta_c - eta(6));           % current surge velocity
v_c = V_c * sin(beta_c - eta(6));           % current sway velocity
nu_r = nu - [u_c v_c 0 0 0 0]';             % relative velocity vector

% Inertia dyadic, volume displacement and draft
nabla = (m+mp)/rho;                               % volume
T = nabla / (2 * Cb_pont * B_pont*L);             % draft
Ig_CG = m * diag([R44^2, R55^2, R66^2]);          % only hull in CG
rg = (m*rg + mp*rp)/(m+mp);                       % CG location corrected for payload
Ig = Ig_CG - m * Smtrx(rg)^2 - mp * Smtrx(rp)^2;  % hull + payload in CO

% Experimental propeller data including lever arms
l1 = -y_pont;                                    % lever arm, left propeller (m)
l2 = y_pont;                                     % lever arm, right propeller (m)
k_pos = 0.02216/2;                               % Positive Bollard, one propeller 
k_neg = 0.01289/2;                               % Negative Bollard, one propeller 
n_max = 300.42; %sqrt((0.5*24.4 * g)/k_pos);     % maximum propeller rev. (rad/s)
n_min = -300.42; %-sqrt((0.5*13.6 * g)/k_neg);   % minimum propeller rev. (rad/s)
F_max = 1000;
F_min = -1000;

% MRB and CRB (Fossen 2021)
I3 = eye(3);
O3 = zeros(3,3);

MRB_CG = [ (m+mp) * I3  O3
           O3           Ig ];
CRB_CG = [ (m+mp) * Smtrx(nu2)         O3
           O3               -Smtrx(Ig*nu2)  ];

H = Hmtrx(rg);              % Transform MRB and CRB from the CG to the CO 
MRB = H' * MRB_CG * H;
CRB = H' * CRB_CG * H;

% disp('MRB =')
% disp(MRB)
% disp('CRB =')
% disp(CRB)

% Hydrodynamic added mass (best practise)
Xudot = -addedMassSurge(m,L,rho);   
Yvdot = -1.5 * m;
Zwdot = -1.0 * m;
Kpdot = -0.2 * Ig(1,1);
Mqdot = -0.8 * Ig(2,2);
Nrdot = -1.7 * Ig(3,3);




MA = -diag([Xudot, Yvdot, Zwdot, Kpdot, Mqdot, Nrdot]);   
CA  = m2c(MA, nu_r);
CA(6,1) = 0; % Assume that the Munk moment in yaw can be neglected
CA(6,2) = 0; % These terms, if nonzero, must be balanced by adding nonlinear damping

% System mass and Coriolis-centripetal matrices
M = MRB + MA;
C = CRB + CA;

% Hydrostatic quantities (Fossen 2021)
Aw_pont = Cw_pont * L * B_pont;    % waterline area, one pontoon 
I_T = 2 * (1/12)*L*B_pont^3 * (6*Cw_pont^3/((1+Cw_pont)*(1+2*Cw_pont)))...
    + 2 * Aw_pont * y_pont^2;
I_L = 0.8 * 2 * (1/12) * B_pont * L^3;
KB = (1/3)*(5*T/2 - 0.5*nabla/(L*B_pont) );
BM_T = I_T/nabla;       % BM values
BM_L = I_L/nabla;
KM_T = KB + BM_T;       % KM values
KM_L = KB + BM_L;
KG = T - rg(3);
GM_T = KM_T - KG;       % GM values
GM_L = KM_L - KG;

G33 = rho * g * (2 * Aw_pont);      % spring stiffness
G44 = rho * g *nabla * GM_T;
G55 = rho * g *nabla * GM_L;

G_CF = diag([0 0 G33 G44 G55 0]);   % spring stiffness matrix in the CF
LCF = -0.2;
%LCF = 0;
H = Hmtrx([LCF 0 0]);               % transform G_CF from the CF to the CO 
G = H' * G_CF * H;

% Natural frequencies
w3 = sqrt( G33/M(3,3) );         
w4 = sqrt( G44/M(4,4) );
w5 = sqrt( G55/M(5,5) );

% Linear damping terms (hydrodynamic derivatives)
    
if nu_r(1) < 1 && nu_r(1) > -1
%     if nu_r(1) < 0.5
%         Xu = -130;
%     else
    Xu = -130;
%    end
else 
     Xu = -51.3;
end

%Xu = -1.5 ;% -51.3;% -775; %(-24.4 * g / Umax);           % specified using the maximum speed  
Yv = -51.3;
Zw = -2 * 0.3 *w3 * M(3,3);      % specified using relative damping factors
Kp = -2 * 0.2 *w4 * M(4,4);
Mq = -2 * 0.4 *w5 * M(5,5);
Nr = -M(6,6) / T_yaw;            % specified using the time constant in T_yaw

% % Control forces and moments - with propeller revolution saturation 
% Thrust = zeros(2,1);
% for i = 1:1:2
%     if n(i) > n_max              % saturation, physical limits
%        n(i) = n_max; 
%     elseif n(i) < n_min
%        n(i) = n_min; 
%     end
%     
%    if n(i) > 0                          
%      Thrust(i) = k_pos * n(i)*abs(n(i));    % positive thrust (N) 
%    else
%      Thrust(i) = k_neg * n(i)*abs(n(i));    % negative thrust (N) 
%    end
% end
% 
% % Control forces and moments
% tau = [Thrust(1) + Thrust(2) 0 0 0 0 -l1 * Thrust(1) - l2 * Thrust(2) ]';

% Control forces and moments - with propeller revolution saturation 

if F_1 > F_max              % saturation, physical limits
  F_1 = F_max; 
elseif F_1 < F_min
  F_1 = F_min; 
end
if F_2 > F_max              % saturation, physical limits
  F_2 = F_max; 
elseif F_1 < F_min
  F_2 = F_min; 
end

% Control forces and moments
tau = [F_1*cos(alpha_1)+F_2*cos(alpha_2) F_1*sin(alpha_1)+F_2*sin(alpha_2) 0 0 0 F_1*y_pont*cos(alpha_1)-F_2*y_pont*cos(alpha_2)]';



% Linear damping using relative velocities + nonlinear yaw damping
Xh = Xu * nu_r(1);
Yh = Yv * nu_r(2); 
Zh = Zw * nu_r(3);
Kh = Kp * nu_r(4);
Mh = Mq * nu_r(5);
%Nh = Nr * (1 + 10 * abs(nu_r(6))) * nu_r(6);
Nh = Nr * (1 + 1 * abs(nu_r(6))) * nu_r(6);


tau_damp = [Xh Yh Zh Kh Mh Nh]';

% Strip theory: cross-flow drag integrals for Yh and Nh
tau_crossflow = crossFlowDrag(L,B_pont,T,nu_r);

% Ballast
g_0 = [0 0 0 0 trim_moment 0]';

% Kinematics
J = eulerang(eta(4),eta(5),eta(6));


%lig = tau + tau_damp + tau_crossflow - C * nu_r - G * eta - g_0   % til at
%finde forces

% Time derivative of the state vector - numerical integration; see ExOtter.m  
xdot = [ M \ ( tau + tau_damp + tau_crossflow - C * nu_r - G * eta - g_0)
         J * nu ];  
     
trim_moment = trim_moment + 0.05 * (trim_setpoint - trim_moment);
U_tot = U;
end

== matlab function system_control/MATLAB Function1 ==
  data: v input; y output
function y = fcn(v)
    if(v == 0.0)
        out = 0.00000000000000000001;
    
    else
        out = v;
    
    end
        

y = out;

== matlab function system_control/vel to thrust (Fx) ==
  data: u_con input; Fx output
function Fx = fcn(u_con)
    x_u = 51.3;
    x_uu = 72.4;
    %knob_2_ms = 0.5144;

    if (u_con < 0)
        k = -1;
    else
        k = 1;
    end
    
    
    
    
    if (u_con == 0)
        T = 0; 
    elseif(abs(u_con) < 1)    
        T = 2*59.7 * abs(u_con) * k;
    else
        %T = 2 * (19.2 *abs(u_con)^2 + 1.5* abs(u_con) + 0)*k;
        T = 2 * (19.2 *abs(u_con)^2 + 1.5* abs(u_con) + 39)*k;
        %T = ((x_u + x_uu * abs(u)) * abs(u))*k;
    end

Fx = T;

== matlab function system_control/vel to thrust (Fy) ==
  data: v input; Fy output
function Fy = fcn(v)

    x_u = 51.3;
    x_uu = 72.4 ;
    %knob_2_ms = 0.5144;
    k_side = 4; % factor for vel sideway

    
    if (v < 0)
        k = -1;
    else
        k = 1;
    end


    T = k_side*((x_u + x_uu * abs(v)) * abs(v))*k;

Fy = T;

== matlab function system_control/Mixer/MATLAB Function ==
  data: F_x input; F_y input; tau input; F_1 output; d input; F_2 output; alpha1 output; alpha2 output; alpha_flag input; alpha_flag_out output; u input; ref_u input; ref_v input; tau_out output
function [F_1, F_2, alpha1, alpha2, alpha_flag_out, tau_out] = fcn(F_x,F_y,tau,d, alpha_flag, u, ref_u, ref_v)    


% limmitting the input signal 
    if (( u < 0.02 && u > -0.02) && (abs(ref_u)< 0.02 && abs(ref_v)< 0.02) && abs(tau) > 0.01)   && alpha_flag == 0
        F_x = 0.0001;
        F_y = 0.0001;
        
    end
    
    
    
    F1 = (0.5000*(F_x*tau + F_x^2*d - tau*(F_x - sqrt(F_x^2 + F_y^2)) - F_x*d*(F_x - sqrt(F_x^2 + F_y^2))))/(F_x*d);
    F2 = -(0.5000*(F_x*tau - F_x^2*d - tau*(F_x - sqrt(F_x^2 + F_y^2)) + F_x*d*(F_x - sqrt(F_x^2 + F_y^2))))/(F_x*d);
    alpha_1 = -2*atan((F_x - sqrt(F_x^2 + F_y^2))/F_y);
    alpha_2 = alpha_1;
    
    % setting the pods when rotating 
    if (F_x == F_y && F_x < 0.001 && F_x > -0.001)  && alpha_flag == 0
        alpha_1 = 0;
        alpha_2 = 0;
    end
    

    
%     disp("================================================")
%     disp("alpha_1 = ")
%     disp(alpha_1)
    
    % sideway: alpha > 70 degrees
    if abs(alpha_1) >= 7*pi/18 && abs(alpha_1) <= 11*pi/18 || abs(alpha_1) <= 25*pi/18 && abs(alpha_1) >= 29*pi/18  
        
        % between +-180 degrees
        if alpha_1 > pi 
            alpha_1 = alpha_1 - 2 * pi;
        elseif alpha_1 < -pi
            alpha_1 = alpha_1 + 2 * pi;
        end       
        % determining the right angle and thrust    
        if alpha_1 > pi/2       %(above 90 degrees)
            alpha_1 = alpha_1 - pi;
        elseif alpha_1 < -pi/2  %(below -90 degrees)
            alpha_1 = alpha_1 + pi;
        end
        
%         disp("==---====---===---===---===---===---===---===---===")
%         disp("alpha_1 = ")
%         disp(alpha_1)
        
%         fprintf("Er HER alpha 1 :---------")
%         disp(alpha_1)
        % if alpha is positvie 
        if alpha_1 >= 0 %|| alpha_1 == -pi/2 %&& alpha_1 < pi/2
            F1 = 1.4618*F_x + 1.0913*tau;
            F2 = (0.5000*F_x - 0.3733*tau - (1.3736*F_x*(2.0634e+18*F_x - 1.5405e+18*tau + 1.4142*sqrt(1.8196e+37*F_x^2 - 2.3394e+37*F_x*F_y + 2.0811e+37*F_x*tau + 8.5155e+36*F_y^2 - 1.7465e+37*F_y*tau + 1.0141e+37*tau^(2))))/(5.6687e+18*F_x - 4.1269e+18*F_y + 4.2320e+18*tau) + (F_y*(2.0634e+18*F_x - 1.5405e+18*tau + 1.4142*sqrt(1.8196e+37*F_x^2 - 2.3394e+37*F_x*F_y + 2.0811e+37*F_x*tau + 8.5155e+36*F_y^2 - 1.7465e+37*F_y*tau + 1.0141e+37*tau^(2))))/(5.6687e+18*F_x - 4.1269e+18*F_y + 4.2320e+18*tau) - (1.0255*tau*(2.0634e+18*F_x - 1.5405e+18*tau + 1.4142*sqrt(1.8196e+37*F_x^2 - 2.3394e+37*F_x*F_y + 2.0811e+37*F_x*tau + 8.5155e+36*F_y^2 - 1.7465e+37*F_y*tau + 1.0141e+37*tau^(2))))/(5.6687e+18*F_x - 4.1269e+18*F_y + 4.2320e+18*tau));
            alpha_1 = 7*pi/18; % 70 degrees
            alpha_2 = 2*atan((2.0634e+18*F_x - 1.5405e+18*tau + 1.4142*sqrt(1.8196e+37*F_x^2 - 2.3394e+37*F_x*F_y + 2.0811e+37*F_x*tau + 8.5155e+36*F_y^2 - 1.7465e+37*F_y*tau + 1.0141e+37*tau^(2)))/(5.6687e+18*F_x - 4.1269e+18*F_y + 4.2320e+18*tau));
%             fprintf("Er HER alpha positiv")
%             fprintf("F1 =")
%             disp(F1)
%             fprintf("F2 =")
%             disp(F2)    
%             fprintf("alpha1 =")
%             disp(alpha_1)
%             fprintf("alpah2 =")
%             disp(alpha_2) 
%             if alpha_2 < 0 && alpha_1 > 0
%                 alpha_2 = pi/2;
%                 F2 = -F2;
%             end
            
        else % if alpha is negative
            F1 = 1.4618*F_x + 1.0913*tau;
            F2 = 3.4268e-19*sqrt(1.8196e+37*F_x^2 + 2.3394e+37*F_x*F_y + 2.0811e+37*F_x*tau + 8.5155e+36*F_y^2 + 1.7465e+37*F_y*tau + 1.0141e+37*tau^(2));
            alpha_1 = -7*pi/18; % -70 degrees
            %alpha_2 = 2*atan((2.0634e+18*F_x - 1.5405e+18*tau + 1.4142*sqrt(1.8196e+37*F_x^2 - 2.3394e+37*F_x*F_y + 2.0811e+37*F_x*tau + 8.5155e+36*F_y^2 - 1.7465e+37*F_y*tau + 1.0141e+37*tau^(2)))/(5.6687e+18*F_x - 4.1269e+18*F_y + 4.2320e+18*tau));
            
            alpha_2 = 2*atan((1.5405e+18*tau - 2.0634e+18*F_x + 1.4142*sqrt(1.8196e+37*F_x^2 + 2.3394e+37*F_x*F_y + 2.0811e+37*F_x*tau + 8.5155e+36*F_y^2 + 1.7465e+37*F_y*tau + 1.0141e+37*tau^(2)))/(5.6687e+18*F_x + 4.1269e+18*F_y + 4.2320e+18*tau));
%             fprintf("Er HER alpha negativ")
%             fprintf("F1 =")
%             disp(F1)
%             fprintf("F2 =")
%             disp(F2)    
%             fprintf("alpha1 =")
%             disp(alpha_1)
%             fprintf("alpah2 =")
%             disp(alpha_2)
        

        end
        
      
        % limitter for angle of pods of 88 degrees
                
        
%         % limmitter and angle determination
%         % angle alpha_2
%         % keeps angle between +-180 degrees
%         if alpha_2 > pi
%             alpha_2 = alpha_2 - 2 * pi;
%         elseif alpha_2 < -pi
%             alpha_2 = alpha_2 + 2 * pi;
%         end       
%         % determining the right angle and thrust    
%         if alpha_2 > pi/2 && alpha_2 < 11*pi/18      %(between 90 and 120 degrees)
%             alpha_2 = alpha_2 - pi;
%             F2 = (-1)*F2;
%         elseif alpha_2 < -pi/2 && alpha_2 > 11*pi/18 %(between -90 and -120 degrees)
%             alpha_2 = alpha_2 + pi;
%             F2 = (-1)*F2;
%         end
% 
%         % limitter for the thrusters for going sideway
%         if abs(F1) > T_max
%             %F1 = T_max;            
%             F1_old = F1;
%             F1 = T_max;
%             F2 = F1/(F1_old/F2);   
%         %elseif F1 < -T_max
%         %    F1 = -T_max;    
%         end
%         if abs(F2) > T_max
%             %F2 = T_max;
%             F2_old = F2;
%             F2 = T_max;
%             F1 = F2/(F2_old/F1);  
%         %elseif F2 < -T_max
%         %   F2 = -T_max;    
%         end
    end

    disp('MIXER F!----------------------------------------------------');
    disp(F1)
    
    % makes shure that the thrusters are straith if no input in surge andsway direction 
    %if F_x == F_y && F_x < 0.001 && F_x > -0.001 && alpha_flag == 0
%     if ((F_x == F_y && F_x < 0.001 && F_x > -0.001) || (abs(u)<0.02 && abs(v) < 0.02))  && alpha_flag == 0
%         alpha_1 = 0;
%         alpha_2 = 0;
%     end
tau_out = tau;
F_1 = F1;
F_2 = F2;
alpha1 = alpha_1;
alpha2 = alpha_2;
alpha_flag_out = alpha_flag;
